simulink model "sim"  (R2025b)
settings: Solver=VariableStepAuto  StartTime=0.0  StopTime=10.0  RelTol=1e-3
settings Model: Creator=flof  LastModifiedBy=flof

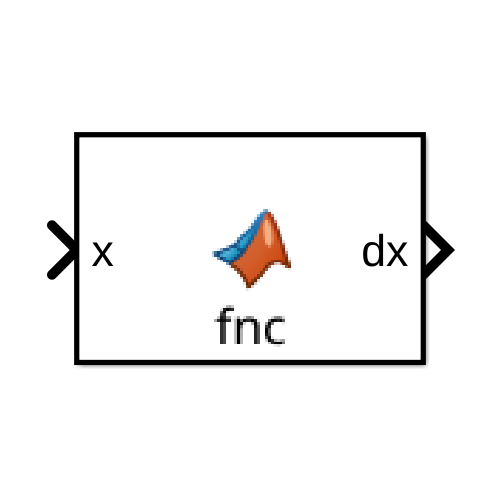
[thumbnail: Simulink's stored preview of the top-level diagram]
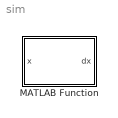
== system sim ==
  MATLAB Function : MATLAB Function  TreatAsAtomicUnit=on

== matlab function sim/MATLAB Function ==
  data: x input; dx output
function dx = fnc(x)

dx = f(x);
